simulink model "Copy_of_Buck_Charger"  (R2023b)
settings: Solver=ode3  StartTime=0.0  StopTime=Ttotal  FixedStep=Tsample  RelTol=1e-3
values from neighbouring files (symbols this model uses):
  A_0 = 1.6882    [Parameters_Buck.m]
  alpha_T = 0.04/100    (= 0.0004)    [Parameters_Buck.m]
  beta_T = -0.29/100    (= -0.0029)    [Parameters_Buck.m]
  Cbat = 33e-6    (= 3.3e-05)    [Parameters_Buck.m]
  Cin = 470e-6    (= 0.00047)    [Parameters_Buck.m]
  delta_x = 1    [Control_Buck.m]
  Ee = 800    [Parameters_Buck.m]
  fmpp = 2e2    (= 200)    [Control_Buck.m]
  I_load = 2.8    [Parameters_Buck.m]
  Ilimit = 60    [Parameters_Buck.m]
  Iscs = Iscs    (= 9.41)    [Parameters_Buck.m]
  Kd0 = (alpha_1^2-2*Wn0(1)*Z0(1)*alpha_1*alpha_2+Wn0(1)^2*alpha_2^2)/K00/(alpha_1^3)    [Control_Buck.m]
  Ki0 = Wn0(1)^2/K00/alpha_1    [Control_Buck.m]
  Kp0 = (2*Wn0(1)*Z0(1)*alpha_1-Wn0(1)^2*alpha_2)/K00/alpha_1^2    [Control_Buck.m]
  L = 470e-6    (= 0.00047)    [Parameters_Buck.m]
  Np = 3    [Parameters_Buck.m]
  qk0 = 11594    [Parameters_Buck.m]
  Rbat = 21.6e-3*4    (= 0.0864)    [Parameters_Buck.m]
  Tau_d0 = alpha_2/alpha_1    [Control_Buck.m]
  Ttotal = 4e-1    (= 0.4)    [Control_Buck.m]
  Vlimit = 55    [Parameters_Buck.m]
  Voc_array = Vocs * Ns*Nss    (= 116.91)    [Parameters_Buck.m]
  Vocs = Vocs/Ns    (= 0.6495)    [Parameters_Buck.m]
  x_init = round(Voc_array*.95)    [Control_Buck.m]
libraries: slpidlib x1
settings Model: Creator=mwxiao  LastModifiedBy=ejom7
settings SolverCC: AlgebraicLoopSolver=TrustRegion
settings DataIOCC: LimitDataPoints=on  SaveFormat=Array  SignalLoggingSaveFormat=ModelDataLogs  ReturnWorkspaceOutputs=off
settings OptimizationCC: ExpressionDepthLimit=2147483647  LifeSpan=inf
settings DebuggingCC: UnderspecifiedInitializationDetection=Classic  MergeDetectMultiDrivingBlocksExec=none  SolverPrmCheckMsg=warning  FcnCallInpInsideContextMsg=warning  UnconnectedInputMsg=warning  UnconnectedOutputMsg=warning  UnconnectedLineMsg=warning  StateNameClashWarn=warning  SFUnexpectedBacktrackingDiag=warning  SFNoUnconditionalDefaultTransitionDiag=warning  SFExecutionAtInitializationDiag=none  ArithmeticOperatorsInVariantConditions=warning
settings HardwareCC: ProdBitPerPointer=32  ProdBitPerSizeT=32  ProdBitPerPtrDiffT=32  ProdLargestAtomicFloat=None  ProdIntDivRoundTo=Undefined  ProdEndianess=Unspecified  ProdWordSize=32  ProdHWDeviceType=32-bit Generic
settings ModelReferenceCC: EnableRefExpFcnMdlSchedulingChecks=on  PropagateSignalLabelsOutOfModel=off
settings SFSimCC: SimUseLocalCustomCode=off  CustomCodeUndefinedFunction=UseInterfaceOnly
settings RTWCC: RTWUseLocalCustomCode=off  DLArmComputeVersion=19.05
settings CodeAppCC: StateflowObjectComments=on
settings GRTTargetCC: TargetLangStandard=C89/C90 (ANSI)  CombineOutputUpdateFcns=off  GRTInterface=on
settings ConfigComp: CovMetricSettings=dw  CovSaveCumulativeToWorkspaceVar=on  CovSaveSingleToWorkspaceVar=on  CovExternalEMLEnable=off

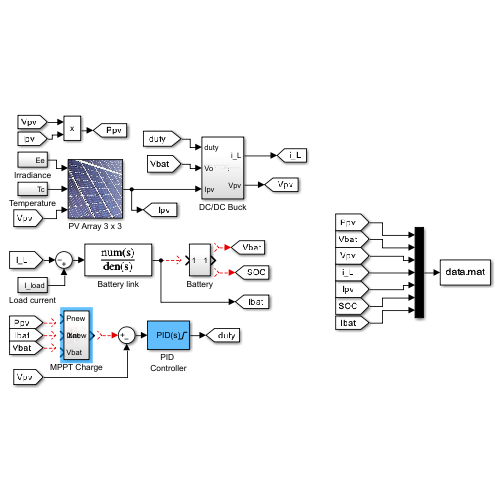
[thumbnail: Simulink's stored preview of the top-level diagram]
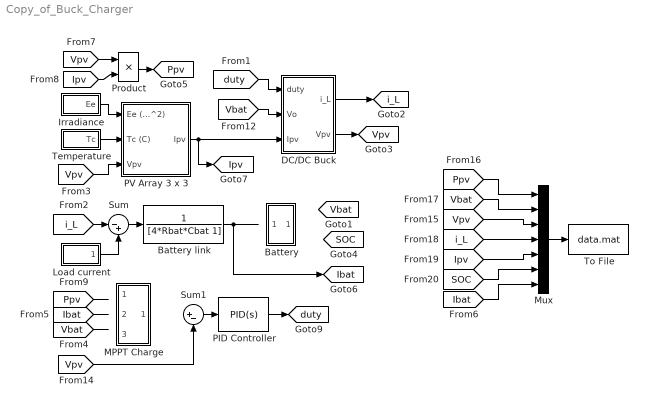
== system Copy_of_Buck_Charger ==
  Battery : Subsystem
  Battery link : TransferFcn  Denominator=[4*Rbat*Cbat 1]
  DC/DC Buck : Subsystem
  Irradiance : Subsystem
  Load current : Subsystem
  MPPT Charge : Subsystem
  Mux : Mux  Inputs=7
  PID Controller : slpidlib/PID Controller  Controller=PID  Form=Parallel  TimeDomain=Continuous-time  UseExternalTs=off  SampleTime=1  IntegratorMethod=Forward Euler  FilterMethod=Forward Euler  ControllerParametersSource=internal  P=Kp0  I=Ki0  UseKiTs=off  D=Kd0  N=1/Tau_d0  UseFilter=on  TunerSelectOption=Transfer Function Based (PID Tuner App)  InitialConditionSource=internal  InitialConditionForIntegrator=0  InitialConditionForFilter=0  DifferentiatorICPrevScaledInput=0  ExternalReset=none  TrackingMode=off  Kt=1  LimitOutput=on  SatLimitsSource=internal  UpperSaturationLimit=.9  LowerSaturationLimit=0  LinearizeAsGain=off  AntiWindupMode=clamping  Kb=1  LimitIntegrator=off  UpperIntegratorSaturationLimit=inf  LowerIntegratorSaturationLimit=-inf  POutMin=[]  POutMax=[]  IOutMin=[]  IOutMax=[]  DOutMin=[]  DOutMax=[]  NOutMin=[]  NOutMax=[]  SumOutMin=[]  SumOutMax=[]  SaturationOutMin=[]  SaturationOutMax=[]  PParamMin=[]  PParamMax=[]  IParamMin=[]  IParamMax=[]  DParamMin=[]  DParamMax=[]  NParamMin=[]  NParamMax=[]  KbParamMin=[]  KbParamMax=[]  KtParamMin=[]  KtParamMax=[]  KbOutMin=[]  KbOutMax=[]  KtOutMin=[]  KtOutMax=[]  IntegratorOutMin=[]  IntegratorOutMax=[]  FilterOutMin=[]  FilterOutMax=[]  SumI1OutMin=[]  SumI1OutMax=[]  SumI2OutMin=[]  SumI2OutMax=[]  SumI3OutMin=[]  SumI3OutMax=[]  SumI4OutMin=[]  SumI4OutMax=[]  SumDOutMin=[]  SumDOutMax=[]  DifferentiatorOutMin=[]  DifferentiatorOutMax=[]  FilterDiffOutCoefMin=[]  FilterDiffOutCoefMax=[]  ReciprocalOutMin=[]  ReciprocalOutMax=[]  SumDenOutMin=[]  SumDenOutMax=[]  SumNumOutMin=[]  SumNumOutMax=[]  DivideOutMin=[]  DivideOutMax=[]  UdiffTsProdOutMin=[]  UdiffTsProdOutMax=[]  NTsProdOutMin=[]  NTsProdOutMax=[]  UintegralTsProdOutMin=[]  UintegralTsProdOutMax=[]  UngainTsProdOutMin=[]  UngainTsProdOutMax=[]  ClampingZeroOutDataTypeStr=Inherit: Inherit via back propagation  ClampingZeroOutMin=[]  ClampingZeroOutMax=[]  FilterDenConstantOutDataTypeStr=Inherit: Inherit via back propagation  FilterDenConstantOutMin=[]  FilterDenConstantOutMax=[]  PCopyOutDataTypeStr=Inherit: Inherit via back propagation  PCopyOutMin=[]  PCopyOutMax=[]  NCopyOutDataTypeStr=Inherit: Inherit via back propagation  NCopyOutMin=[]  NCopyOutMax=[]  IntegratorContinuousStateAttributes=''  IntegratorStateMustResolveToSignalObject=off  IntegratorRTWStateStorageClass=Auto  FilterContinuousStateAttributes=''  FilterStateMustResolveToSignalObject=off  FilterRTWStateStorageClass=Auto  ParallelPVariant=InternalParameters  IdealPVariant=Disabled  IVariant=InternalParameters  DVariant=InternalParameters  IntegratorVariant=Continuous  SatVariant=Enabled  AWVariant=ContClampingParallel  PCopyVariant=Disabled  TRVariant=Disabled  FdbkBlocksVariant=Forward  IdealPFdbkVariant=Disabled  SatFdbkVariant=Disabled  DerivativeFilterVariant=ContFilter  NVariant=InternalParameters  NCopyVariant=Disabled  FilterICVariant=InternalICsFilter  IntegratorICVariant=InternalICs  ExternalResetVariant=Disabled  TRSumVariant=Passthrough  SumFdbkVariant=Disabled  SumVariant=Sum_PID  TsampFilterVariant=InternalTs  TsampNgainVariant=Passthrough  TsampIntegralVariant=Disabled_SignalSpec  ExternalSaturationOutDataTypeStr=Inherit: Same as second input
  PV Array 3 x 3 : Subsystem
      mask Display: image(imread('icon01.jpg'))
  Product : Product  RndMeth=Zero
  Sum : Sum  Inputs=|-+
  Sum1 : Sum  Inputs=|+-
  Temperature : Subsystem
  To File : ToFile  Filename=data.mat  SaveFormat=Timeseries
  tag scope: Ibat=global, Ipv=global, Ppv=global, SOC=global, Vbat=global, Vpv=global, duty=global, i_L=global
  wires:
  DC/DC Buck/1(i_L) -> [i_L]
  DC/DC Buck/2(Vpv) -> [Vpv]
  Irradiance/1(Ee) -> PV Array 3 x 3/1(Ee (W/m^2))
  Temperature/1(Tc) -> PV Array 3 x 3/2(Tc (C))
  [Vpv] -> PV Array 3 x 3/3(Vpv)
  PV Array 3 x 3/1(Ipv) -> DC/DC Buck/3(Ipv), [Ipv]
  Product/1 -> [Ppv]
  [Vpv] -> Product/1
  [Ipv] -> Product/2
  ? -> Sum1/1
  [Vpv] -> Sum1/2
  Sum1/1 -> PID Controller/1
  [Ppv] -> Mux/1
  [Vbat] -> Mux/2
  [Vpv] -> Mux/3
  [Ipv] -> Mux/5
  [SOC] -> Mux/6
  Load current/1(I_load) -> Sum/2
  Battery link/1 -> [Ibat]
  Sum/1 -> Battery link/1
  ? -> [Vbat]
  ? -> [SOC]
  [i_L] -> Sum/1
  [Ppv] -> ?
  [Vbat] -> ?
  [Ibat] -> ?
  [Ibat] -> Mux/7
  [i_L] -> Mux/4
  Mux/1 -> To File/1
  PID Controller/1 -> [duty]
  [duty] -> DC/DC Buck/1(duty)
  [Vbat] -> DC/DC Buck/2(Vo)

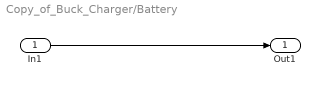
== system Copy_of_Buck_Charger/Battery ==
  In1 : Inport
  Out1 : Outport
  wires:
  In1/1 -> Out1/1

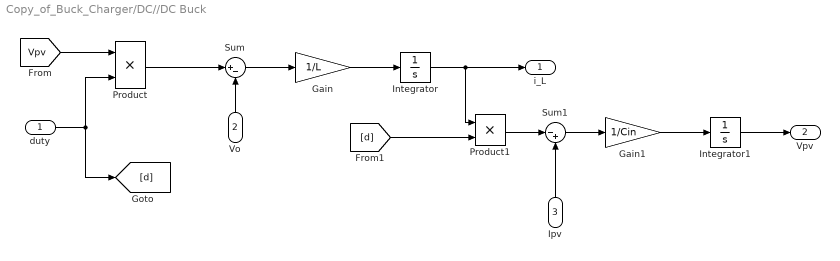
== system Copy_of_Buck_Charger/DC//DC Buck ==
  duty : Inport
  Vo : Inport  Port=2
  Ipv : Inport  Port=3
  Gain : Gain  Gain=1/L
  Gain1 : Gain  Gain=1/Cin
  Integrator : Integrator  LimitOutput=on  LowerSaturationLimit=0
  Integrator1 : Integrator  InitialCondition=Voc_array  LimitOutput=on  LowerSaturationLimit=0
  Product : Product
  Product1 : Product
  Sum : Sum  Inputs=|+-
  Sum1 : Sum  Inputs=|-+
  i_L : Outport
  Vpv : Outport  Port=2
  wires:
  duty/1 -> [d], Product/2
  [Vpv] -> Product/1
  Product/1 -> Sum/1
  Vo/1 -> Sum/2
  Sum/1 -> Gain/1
  Gain/1 -> Integrator/1
  Integrator/1 -> Product1/1, i_L/1
  [d] -> Product1/2
  Product1/1 -> Sum1/1
  Ipv/1 -> Sum1/2
  Gain1/1 -> Integrator1/1
  Integrator1/1 -> Vpv/1
  Sum1/1 -> Gain1/1

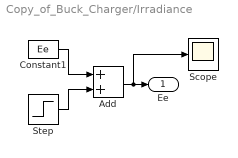
== system Copy_of_Buck_Charger/Irradiance ==
  Add : Sum
  Constant1 : Constant  Value=Ee
  Scope : Scope
  Step : Step  Time=Ttotal/2  After=-Ee/2  SampleTime=0
  Ee : Outport
  wires:
  Constant1/1 -> Add/1
  Step/1 -> Add/2
  Add/1 -> Ee/1, Scope/1

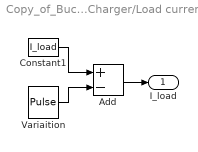
== system Copy_of_Buck_Charger/Load current ==
  Add : Sum  Inputs=+-
  Constant1 : Constant  Value=I_load
  Variaition : DiscretePulseGenerator  PulseType=Time based  Amplitude=0  Period=15e-3  PulseWidth=50  PhaseDelay=Ttotal/2
  I_load : Outport
  wires:
  Constant1/1 -> Add/1
  Variaition/1 -> Add/2
  Add/1 -> I_load/1

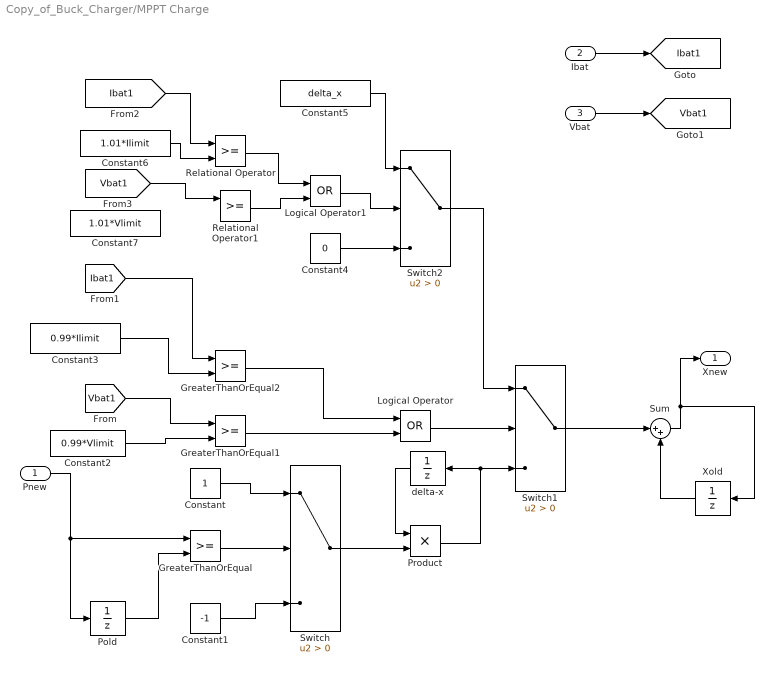
== system Copy_of_Buck_Charger/MPPT Charge ==
  Pnew : Inport  SampleTime=1/fmpp
  Ibat : Inport  Port=2  SampleTime=1/fmpp
  Vbat : Inport  Port=3  SampleTime=1/fmpp
  Constant : Constant  SampleTime=1/fmpp
  Constant1 : Constant  Value=-1  SampleTime=1/fmpp
  Constant2 : Constant  Value=0.99*Vlimit  SampleTime=1/fmpp
  Constant3 : Constant  Value=0.99*Ilimit  SampleTime=1/fmpp
  Constant4 : Constant  Value=0  SampleTime=1/fmpp
  Constant5 : Constant  Value=delta_x  SampleTime=1/fmpp
  Constant6 : Constant  Value=1.01*Ilimit  SampleTime=1/fmpp
  Constant7 : Constant  Value=1.01*Vlimit  SampleTime=1/fmpp
  GreaterThanOrEqual : RelationalOperator  OutDataTypeStr=boolean  RndMeth=Simplest  InputSameDT=off
  GreaterThanOrEqual1 : RelationalOperator  OutDataTypeStr=boolean  RndMeth=Simplest  InputSameDT=off
  GreaterThanOrEqual2 : RelationalOperator  OutDataTypeStr=boolean  RndMeth=Simplest  InputSameDT=off
  Logical Operator : Logic  Operator=OR  AllPortsSameDT=off  OutDataTypeStr=boolean
  Logical Operator1 : Logic  Operator=OR  AllPortsSameDT=off  OutDataTypeStr=boolean
  Pold : UnitDelay  InitialCondition=1e3  SampleTime=1/fmpp  HasFrameUpgradeWarning=on
  Product : Product
  Relational Operator : RelationalOperator  OutDataTypeStr=boolean  RndMeth=Simplest  InputSameDT=off
  Relational Operator1 : RelationalOperator  OutDataTypeStr=boolean  RndMeth=Simplest  InputSameDT=off
  Sum : Sum  Inputs=|++
  Switch : Switch  Criteria=u2 > Threshold  SaturateOnIntegerOverflow=off  InputSameDT=off
  Switch1 : Switch  Criteria=u2 > Threshold  SaturateOnIntegerOverflow=off  InputSameDT=off
  Switch2 : Switch  Criteria=u2 > Threshold  SaturateOnIntegerOverflow=off  InputSameDT=off
  Xold : UnitDelay  InitialCondition=x_init  SampleTime=1/fmpp  HasFrameUpgradeWarning=on
  delta-x : UnitDelay  InitialCondition=delta_x  SampleTime=1/fmpp  HasFrameUpgradeWarning=on
  Xnew : Outport  SampleTime=1/fmpp
  tag scope: Ibat1=global, Vbat1=global
  wires:
  Pnew/1 -> GreaterThanOrEqual/1, Pold/1
  Pold/1 -> GreaterThanOrEqual/2
  Constant/1 -> Switch/1
  GreaterThanOrEqual/1 -> Switch/2
  Constant1/1 -> Switch/3
  Switch/1 -> Product/2
  delta-x/1 -> Product/1
  Product/1 -> delta-x/1, Switch1/3
  Logical Operator/1 -> Switch1/2
  GreaterThanOrEqual1/1 -> Logical Operator/2
  GreaterThanOrEqual2/1 -> Logical Operator/1
  Constant2/1 -> GreaterThanOrEqual1/2
  [Vbat1] -> GreaterThanOrEqual1/1
  Constant3/1 -> GreaterThanOrEqual2/2
  [Ibat1] -> GreaterThanOrEqual2/1
  Switch2/1 -> Switch1/1
  Constant4/1 -> Switch2/3
  Constant5/1 -> Switch2/1
  Logical Operator1/1 -> Switch2/2
  Relational Operator/1 -> Logical Operator1/1
  Relational Operator1/1 -> Logical Operator1/2
  [Ibat1] -> Relational Operator/1
  Constant6/1 -> Relational Operator/2
  [Vbat1] -> Relational Operator1/1
  Ibat/1 -> [Ibat1]
  Vbat/1 -> [Vbat1]
  Switch1/1 -> Sum/1
  Sum/1 -> Xold/1, Xnew/1
  Xold/1 -> Sum/2

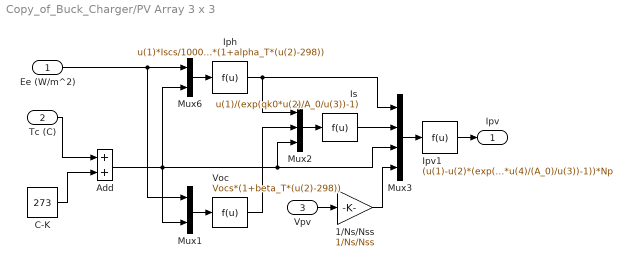
== system Copy_of_Buck_Charger/PV Array 3 x 3 ==
  Ee (W/m^2) : Inport
  Tc (C) : Inport  Port=2
  Vpv : Inport  Port=3
  1/Ns/Nss : Gain  Gain=1/Ns/Nss
  Add : Sum
  C-K : Constant  Value=273
  Iph : Fcn  Expr=u(1)*Iscs/1000*(1+alpha_T*(u(2)-298))
  Ipv1 : Fcn  Expr=(u(1)-u(2)*(exp(qk0*u(4)/(A_0)/u(3))-1))*Np
  Is : Fcn  Expr=u(1)/(exp(qk0*u(2)/A_0/u(3))-1)
  Mux1 : Mux  Inputs=2
  Mux2 : Mux  Inputs=3
  Mux3 : Mux
  Mux6 : Mux  Inputs=2
  Voc : Fcn  Expr=Vocs*(1+beta_T*(u(2)-298))
  Ipv : Outport
  wires:
  Mux6/1 -> Iph/1
  Ee (W/m^2)/1 -> Mux6/1, Mux1/1
  Mux1/1 -> Voc/1
  Mux2/1 -> Is/1
  Iph/1 -> Mux2/1, Mux3/1
  Voc/1 -> Mux2/2
  Mux3/1 -> Ipv1/1
  Is/1 -> Mux3/2
  Vpv/1 -> 1/Ns/Nss/1
  Ipv1/1 -> Ipv/1
  Tc (C)/1 -> Add/1
  Add/1 -> Mux6/2, Mux1/2, Mux3/3, Mux2/3
  C-K/1 -> Add/2
  1/Ns/Nss/1 -> Mux3/4

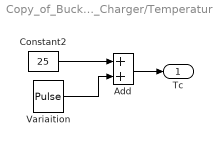
== system Copy_of_Buck_Charger/Temperature ==
  Add : Sum
  Constant2 : Constant  Value=25
  Variaition : DiscretePulseGenerator  PulseType=Time based  Amplitude=0  Period=20e-3  PulseWidth=50  PhaseDelay=Ttotal/4
  Tc : Outport
  wires:
  Constant2/1 -> Add/1
  Variaition/1 -> Add/2
  Add/1 -> Tc/1
